simulink model "target_model"  (R2020b)
settings: Solver=VariableStepAuto  StartTime=0.0  StopTime=10.0  RelTol=1e-3
libraries: arduinolib x9, pid_lib x1
settings Model: Creator=priyankdubey  LastModifiedBy=priyankdubey

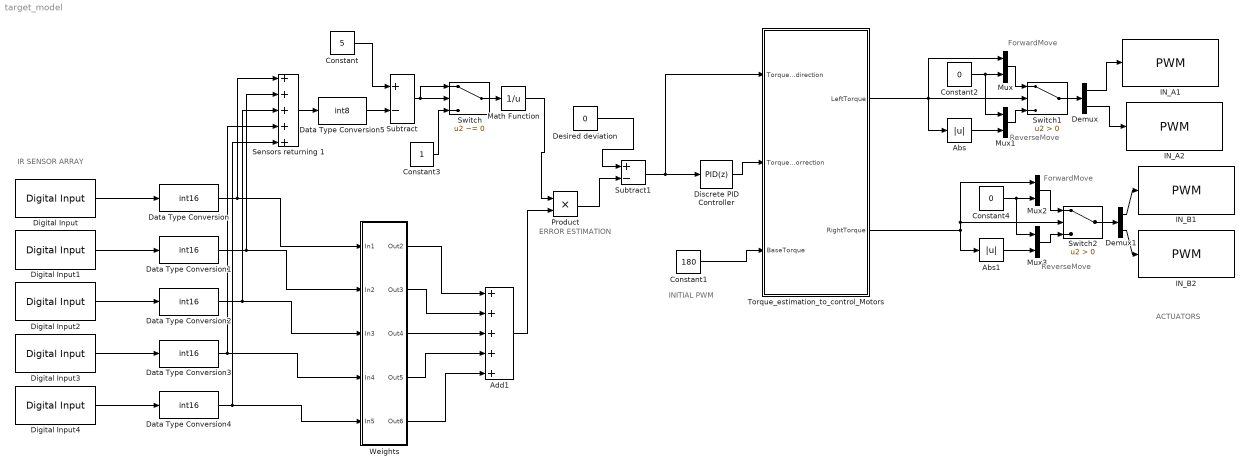
== system target_model ==
  note: ERROR ESTIMATION
  note: INITIAL PWM
  note: ACTUATORS
  note: IR SENSOR ARRAY
  note: ForwardMove
  note: ReverseMove
  note: ReverseMove
  note: ForwardMove
  Abs : Abs  OutDataTypeStr=int16  RndMeth=Round
  Abs1 : Abs  OutDataTypeStr=int16  RndMeth=Round
  Add1 : Sum  Inputs=+++++  AccumDataTypeStr=int8  OutDataTypeStr=int8
  Constant : Constant  Value=5  OutDataTypeStr=int8
  Constant1 : Constant  Value=180
  Constant2 : Constant  Value=0  OutDataTypeStr=int16
  Constant3 : Constant  OutDataTypeStr=int8
  Constant4 : Constant  Value=0  OutDataTypeStr=int16
  Data Type Conversion{,1..4} (5 alike) : DataTypeConversion  OutDataTypeStr=int16
  Data Type Conversion5 : DataTypeConversion  OutDataTypeStr=int8
  Demux : Demux  Outputs=2
  Demux1 : Demux  Outputs=2
  Desired deviation : Constant  Value=0  OutDataTypeStr=int8
  Digital Input{,1..4} (5 alike) : arduinolib/Digital Input  pinNumber=8  mode=Default  Direction=input  SampleTime=0.1  blockPlatform=arduino
  Discrete PID Controller : pid_lib/PID Controller  Controller=PID  Form=Parallel  TimeDomain=Discrete-time  UseExternalTs=off  SampleTime=-1  IntegratorMethod=Forward Euler  FilterMethod=Forward Euler  ControllerParametersSource=internal  P=35  I=15  D=0.005  UseFilter=off  N=60  TunerSelectOption=Transfer Function Based (PID Tuner App)  InitialConditionSource=internal  InitialConditionForIntegrator=0  InitialConditionForFilter=0  DifferentiatorICPrevScaledInput=0  ExternalReset=none  TrackingMode=off  Kt=1  LimitOutput=off  SatLimitsSource=internal  UpperSaturationLimit=inf  LowerSaturationLimit=-inf  LinearizeAsGain=on  AntiWindupMode=none  Kb=1  RndMeth=Round  PGainOutDataTypeStr=int16  PProdOutDataTypeStr=int16  POutMin=[]  POutMax=[]  IGainOutDataTypeStr=int16  IProdOutDataTypeStr=int16  IOutMin=[]  IOutMax=[]  DGainOutDataTypeStr=int16  DProdOutDataTypeStr=int16  DOutMin=[]  DOutMax=[]  NGainOutDataTypeStr=int8  NProdOutDataTypeStr=int8  NOutMin=[]  NOutMax=[]  SumOutDataTypeStr=int16  SumOutMin=[]  SumOutMax=[]  SaturationOutMin=[]  SaturationOutMax=[]  PParamDataTypeStr=int16  PParamMin=[]  PParamMax=[]  IParamDataTypeStr=int16  IParamMin=[]  IParamMax=[]  DParamDataTypeStr=int16  DParamMin=[]  DParamMax=[]  NParamDataTypeStr=int8  NParamMin=[]  NParamMax=[]  KbParamMin=[]  KbParamMax=[]  KtParamMin=[]  KtParamMax=[]  KbOutMin=[]  KbOutMax=[]  KtOutMin=[]  KtOutMax=[]  IntegratorOutDataTypeStr=int16  IntegratorOutMin=[]  IntegratorOutMax=[]  FilterOutDataTypeStr=int8  FilterOutMin=[]  FilterOutMax=[]  SumI1OutMin=[]  SumI1OutMax=[]  SumI2OutMin=[]  SumI2OutMax=[]  SumI3OutMin=[]  SumI3OutMax=[]  SumI4OutMin=[]  SumI4OutMax=[]  SumDOutDataTypeStr=int8  SumDOutMin=[]  SumDOutMax=[]  SumAccumDataTypeStr=int16  SumDAccumDataTypeStr=int8  DifferentiatorOutMin=[]  DifferentiatorOutMax=[]  FilterDiffOutCoefMin=[]  FilterDiffOutCoefMax=[]  ReciprocalOutMin=[]  ReciprocalOutMax=[]  SumDenOutMin=[]  SumDenOutMax=[]  SumNumOutMin=[]  SumNumOutMax=[]  DivideOutMin=[]  DivideOutMax=[]  UdiffTsProdOutMin=[]  UdiffTsProdOutMax=[]  NTsProdOutMin=[]  NTsProdOutMax=[]  UintegralTsProdOutMin=[]  UintegralTsProdOutMax=[]  UngainTsProdOutMin=[]  UngainTsProdOutMax=[]  IntegratorContinuousStateAttributes=''  IntegratorStateMustResolveToSignalObject=off  IntegratorRTWStateStorageClass=Auto  FilterContinuousStateAttributes=''  FilterStateMustResolveToSignalObject=off  FilterRTWStateStorageClass=Auto  ParallelPVariant=InternalParameters  IdealPVariant=Disabled  IVariant=InternalParameters  DVariant=InternalParameters  IntegratorVariant=Discrete  SatVariant=Disabled  AWVariant=Passthrough  PCopyVariant=Disabled  TRVariant=Disabled  FdbkBlocksVariant=Forward  IdealPFdbkVariant=Disabled  SatFdbkVariant=Disabled  DerivativeFilterVariant=Differentiator  NVariant=Passthrough  NCopyVariant=Disabled_SignalSpec  FilterICVariant=InternalICsDifferentiator  IntegratorICVariant=InternalICs  ExternalResetVariant=Disabled  TRSumVariant=Passthrough  SumFdbkVariant=Disabled  SumVariant=Sum_PID  TsampFilterVariant=InternalTs  TsampNgainVariant=Passthrough  TsampIntegralVariant=Passthrough  ExternalSaturationOutDataTypeStr=Inherit: Same as second input
  IN_A1 : arduinolib/PWM  pinNumber=6  frequencyType=Default  desiredFrequency=490.2  achievableFrequency=490.2
  IN_A2 : arduinolib/PWM  pinNumber=5  frequencyType=Default  desiredFrequency=490.2  achievableFrequency=490.2
  IN_B1 : arduinolib/PWM  pinNumber=10  frequencyType=Default  desiredFrequency=490.2  achievableFrequency=490.2
  IN_B2 : arduinolib/PWM  pinNumber=9  frequencyType=Default  desiredFrequency=490.2  achievableFrequency=490.2
  Math Function : Math  Operator=reciprocal  SignedPower=on  SaturateOnIntegerOverflow=on  OutDataTypeStr=Inherit: Inherit via internal rule
  Mux{,1..3} (4 alike) : Mux  Inputs=2
  Product : Product  OutDataTypeStr=int8  RndMeth=Round
  Sensors returning 1 : Sum  Inputs=+++++  AccumDataTypeStr=int8  OutDataTypeStr=int8
  Subtract : Sum  Inputs=+-  AccumDataTypeStr=int8  OutDataTypeStr=int8  RndMeth=Round
  Subtract1 : Sum  Inputs=+-  AccumDataTypeStr=int8  OutDataTypeStr=int8
  Switch : Switch  Criteria=u2 ~= 0  Threshold=0.0001
  Switch1 : Switch  Criteria=u2 > Threshold
  Switch2 : Switch  Criteria=u2 > Threshold
  Torque_estimation_to_control_Motors : Stateflow chart  TreatAsAtomicUnit=on
  Weights : Subsystem
  wires:
  Constant3/1 -> Switch/3
  Data Type Conversion4/1 -> Weights/5(In5), Sensors returning 1/5
  Subtract/1 -> Switch/1, Switch/2
  Add1/1 -> Product/2
  Weights/2(Out3) -> Add1/2
  Desired deviation/1 -> Subtract1/1
  Weights/1(Out2) -> Add1/1
  Subtract1/1 -> Torque_estimation_to_control_Motors/1(Torque_direction), Discrete PID Controller/1
  Data Type Conversion2/1 -> Weights/3(In3), Sensors returning 1/3
  Discrete PID Controller/1 -> Torque_estimation_to_control_Motors/2(Torque_correction)
  Switch/1 -> Math Function/1
  Sensors returning 1/1 -> Data Type Conversion5/1
  Constant/1 -> Subtract/1
  Digital Input4/1 -> Data Type Conversion4/1
  Weights/5(Out6) -> Add1/5
  Constant1/1 -> Torque_estimation_to_control_Motors/3(BaseTorque)
  Math Function/1 -> Product/1
  Weights/4(Out5) -> Add1/4
  Data Type Conversion5/1 -> Subtract/2
  Digital Input1/1 -> Data Type Conversion1/1
  Digital Input/1 -> Data Type Conversion/1
  Digital Input2/1 -> Data Type Conversion2/1
  Weights/3(Out4) -> Add1/3
  Torque_estimation_to_control_Motors/2(RightTorque) -> Abs1/1, Mux2/1, Switch2/2
  Digital Input3/1 -> Data Type Conversion3/1
  Product/1 -> Subtract1/2
  Data Type Conversion3/1 -> Weights/4(In4), Sensors returning 1/4
  Data Type Conversion/1 -> Weights/1(In1), Sensors returning 1/1
  Abs/1 -> Mux1/2
  Data Type Conversion1/1 -> Weights/2(In2), Sensors returning 1/2
  Torque_estimation_to_control_Motors/1(LeftTorque) -> Abs/1, Mux/1, Switch1/2
  Switch1/1 -> Demux/1
  Demux1/1 -> IN_B1/1
  Demux/2 -> IN_A2/1
  Mux/1 -> Switch1/1
  Switch2/1 -> Demux1/1
  Constant4/1 -> Mux2/2, Mux3/1
  Demux1/2 -> IN_B2/1
  Demux/1 -> IN_A1/1
  Abs1/1 -> Mux3/2
  Constant2/1 -> Mux/2, Mux1/1
  Mux3/1 -> Switch2/3
  Mux1/1 -> Switch1/3
  Mux2/1 -> Switch2/1

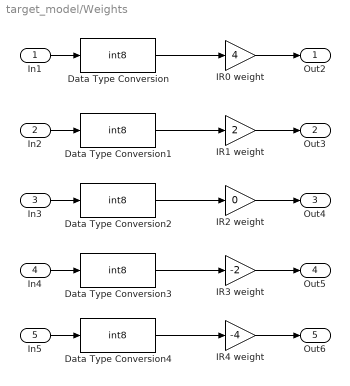
== system target_model/Weights ==
  In1 : Inport
  In2 : Inport  Port=2
  In3 : Inport  Port=3
  In4 : Inport  Port=4
  In5 : Inport  Port=5
  Data Type Conversion{,1..4} (5 alike) : DataTypeConversion  OutDataTypeStr=int8
  IR0 weight : Gain  Gain=4  OutDataTypeStr=int8
  IR1 weight : Gain  Gain=2  OutDataTypeStr=int8
  IR2 weight : Gain  Gain=0  OutDataTypeStr=int8
  IR3 weight : Gain  Gain=-2  OutDataTypeStr=int8
  IR4 weight : Gain  Gain=-4  OutDataTypeStr=int8
  Out2 : Outport  VectorParamsAs1DForOutWhenUnconnected=off
  Out3 : Outport  Port=2  VectorParamsAs1DForOutWhenUnconnected=off
  Out4 : Outport  Port=3  VectorParamsAs1DForOutWhenUnconnected=off
  Out5 : Outport  Port=4  VectorParamsAs1DForOutWhenUnconnected=off
  Out6 : Outport  Port=5  VectorParamsAs1DForOutWhenUnconnected=off
  wires:
  In2/1 -> Data Type Conversion1/1
  In1/1 -> Data Type Conversion/1
  In5/1 -> Data Type Conversion4/1
  In3/1 -> Data Type Conversion2/1
  In4/1 -> Data Type Conversion3/1
  IR0 weight/1 -> Out2/1
  IR2 weight/1 -> Out4/1
  IR1 weight/1 -> Out3/1
  IR3 weight/1 -> Out5/1
  IR4 weight/1 -> Out6/1
  Data Type Conversion3/1 -> IR3 weight/1
  Data Type Conversion4/1 -> IR4 weight/1
  Data Type Conversion2/1 -> IR2 weight/1
  Data Type Conversion1/1 -> IR1 weight/1
  Data Type Conversion/1 -> IR0 weight/1

== stateflow chart target_model/Torque_estimation_to_control_Motors ==
  state GoStraight
    entry:
    LeftTorque = int16(15)+BaseTorque;
    RightTorque = int16(15)+BaseTorque;
  state TurnLeft
    entry:
    LeftTorque = BaseTorque - abs(Torque_correction);
    RightTorque = BaseTorque + abs(Torque_correction);
  state TurnRight
    entry:
    LeftTorque = BaseTorque + abs(Torque_correction);
    RightTorque = BaseTorque - abs(Torque_correction);
  (default) -> GoStraight
  GoStraight -> TurnRight [order 2] : [Torque_direction > 0]
  GoStraight -> TurnLeft [order 1] : [Torque_direction < 0]
  TurnRight -> GoStraight [order 1] : [Torque_direction == 0]
  TurnLeft -> GoStraight [order 2] : [Torque_direction == 0]
  TurnLeft -> TurnRight [order 1] : [Torque_direction > 0]
  TurnRight -> TurnLeft [order 2] : [Torque_direction < 0]
  data: Torque_direction input int8; Torque_correction input int16; BaseTorque input int16; LeftTorque output int16 [0..255]; RightTorque output int16 [0..255]
